simulink model "Module6"  (R2013a)
settings: Solver=FixedStepDiscrete  StartTime=0.0  StopTime=0.05  FixedStep=1e-5  RelTol=1e-3
undefined symbols (not defined in the file or in its folder): get
libraries: dspxfrm3 x2, dspsnks4 x2, dspsigops x2
settings Model: Creator=Lee  LastModifiedBy=cory

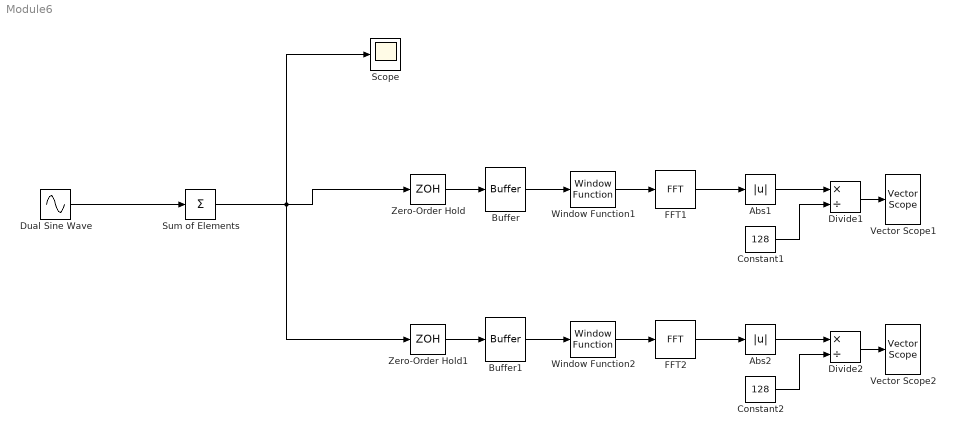
== system Module6 ==
  Abs1 : Abs
  Abs2 : Abs
  Buffer : Buffer  N=128  TreatMby1Signals=One channel
  Buffer1 : Buffer  N=128  TreatMby1Signals=One channel
  Constant1 : Constant  Value=128
  Constant2 : Constant  Value=128
  Divide1 : Product  Inputs=*/
  Divide2 : Product  Inputs=*/
  Dual Sine Wave : Sin  Amplitude=[1, 1]  Bias=[0, 0]  Frequency=2*pi*[0.9, 1.1]*1e3  Phase=[0, 0]  SampleTime=0
  FFT1 : dspxfrm3/FFT  CompMethod=Table lookup  TableOpt=NEW  TableOptActive=Speed  BitRevOrder=off  InheritFFTLength=on  FFTLength=64  RowConvenienceOn=on  FFTImplementation=Auto  SkipNorm=off  firstCoeffDataTypeStr=Inherit: Same word length as input  firstCoeffLastDataTypeStr=Inherit: Same word length as input  outputMin=[]  outputMax=[]  roundingMode=Floor  overflowMode=off
  FFT2 : dspxfrm3/FFT  CompMethod=Table lookup  TableOpt=NEW  TableOptActive=Speed  BitRevOrder=off  InheritFFTLength=on  FFTLength=64  RowConvenienceOn=on  FFTImplementation=Auto  SkipNorm=off  firstCoeffDataTypeStr=Inherit: Same word length as input  firstCoeffLastDataTypeStr=Inherit: Same word length as input  outputMin=[]  outputMax=[]  roundingMode=Floor  overflowMode=off
  Scope : Scope
      settings: TimeRange=0.09052471482889736  YMin=-0.90625  YMax=1.15625
  Sum of Elements : Sum  Inputs=+
  Vector Scope1 : dspsnks4/Vector Scope  ScopeProperties=on  Domain=Frequency  HorizSpan=1  DisplayProperties=off  AxisGrid=on  Memory=off  FrameNumber=on  AxisLegend=off  AxisZoom=off  OpenScopeAtSimStart=on  OpenScopeImmediately=off  FigPos=get(0,'defaultfigureposition')  AxisProperties=off  XUnits=Hertz  XRange=[0...Fs/2]  InheritXIncr=on  XIncr=1  XLabel=Time  XLimit=Auto  XMin=0  XMax=1  XStart=0  YUnits=dB  YLabel=Amplitude  LineProperties=off  XAxisParamsVer=6.9
      settings: YMin=-100  YMax=1
  Vector Scope2 : dspsnks4/Vector Scope  ScopeProperties=on  Domain=Frequency  HorizSpan=1  DisplayProperties=off  AxisGrid=on  Memory=off  FrameNumber=on  AxisLegend=off  AxisZoom=off  OpenScopeAtSimStart=on  OpenScopeImmediately=off  FigPos=get(0,'defaultfigureposition')  AxisProperties=off  XUnits=Hertz  XRange=[0...Fs/2]  InheritXIncr=on  XIncr=1  XLabel=Time  XLimit=Auto  XMin=0  XMax=1  XStart=0  YUnits=dB  YLabel=Amplitude  LineProperties=off  XAxisParamsVer=6.9
      settings: YMin=-100  YMax=1
  Window Function1 : dspsigops/Window Function  winmode=Apply window to input  wintype=Hann  sampmode=Continuous  samptime=1  N=64  Rs=50  beta=10  winsamp=Symmetric  UserWindow=hamming  OptParams=off  UserParams={'symmetric'}  RowConvenienceOn=on  dataType=double  isSigned=on  wordLen=16  udDataType=sfix(16)  fracBitsMode=Best precision  numFracBits=15  roundingMode=Floor  overflowMode=off  numSidelobes=4  sidelobeLevel=-30
  Window Function2 : dspsigops/Window Function  winmode=Apply window to input  wintype=Hann  sampmode=Continuous  samptime=1  N=64  Rs=50  beta=10  winsamp=Symmetric  UserWindow=hamming  OptParams=off  UserParams={'symmetric'}  RowConvenienceOn=on  dataType=double  isSigned=on  wordLen=16  udDataType=sfix(16)  fracBitsMode=Best precision  numFracBits=15  roundingMode=Floor  overflowMode=off  numSidelobes=4  sidelobeLevel=-30
  Zero-Order Hold : ZeroOrderHold  SampleTime=5e-5
  Zero-Order Hold1 : ZeroOrderHold  SampleTime=0.0002
  wires:
  Zero-Order Hold/1 -> Buffer/1
  FFT1/1 -> Abs1/1
  Constant1/1 -> Divide1/2
  Abs1/1 -> Divide1/1
  Divide1/1 -> Vector Scope1/1
  Buffer/1 -> Window Function1/1
  Window Function1/1 -> FFT1/1
  Dual Sine Wave/1 -> Sum of Elements/1
  Zero-Order Hold1/1 -> Buffer1/1
  FFT2/1 -> Abs2/1
  Constant2/1 -> Divide2/2
  Abs2/1 -> Divide2/1
  Divide2/1 -> Vector Scope2/1
  Buffer1/1 -> Window Function2/1
  Window Function2/1 -> FFT2/1
  Sum of Elements/1 -> Zero-Order Hold1/1, Scope/1, Zero-Order Hold/1
